simulink library "BAMLIB564xL"  (Simulink 7.3)
settings: Solver=FixedStepDiscrete  StartTime=0.0  StopTime=10.0  RelTol=1e-3
undefined symbols (not defined in the file or in its folder): CoefBuf, Kx, Ky, Order, ps32Table, s32A1, s32A2, s32ArgDcBusMsr, s32B0, s32B1, s32B2, s32C1, s32CC1, s32CC2, s32HystOff, s32HystOn, s32IntegGain, s32Kd, s32Kq, s32Lim, s32LowerLim, s32LowerLimit, s32MidId, s32MidIdx, s32ModIndex, s32OutValOff, s32OutValOn, s32PropGain, s32RampDown, s32RampUp, s32ShamOffset, s32ShamOffset1, s32ShamOffset2, s32UpperLim, s32UpperLimit, ThetaAdj, u16NSamples
(part 2 of 2)

== system BAMLIB564xL/General Functions/GFLIB_Sin ==
  note: ---------------------------------------------------------------------------------------------------------------------------------------------------------------------------------------------------
  s32In : Inport  OutDataType=fixdt(1, 16)  OutScaling=2^0
  GFLIB_Sin_SF_FLT : S-Function  FunctionName=GFLIB_Sin_SF_FLT  EnableBusSupport=off
  copyright : Subsystem
      mask Display: text(10,90,'FILE:');text(10,75,'DESRIPTION:')text(10,60,'COPYRIGHT:')text(10,45,'VERSION:')text(10,30,'DATE:')text(10,15,'AUTHOR:')
  copyright2 : Subsystem
      mask Display: text(10,90,'GFLIB_Sin_BAM_FLT.mdl');text(10,75,'sin');text(10,60,'Freescale')text(10,45,'0.1');text(10,30,'29-Sep-2010');text(10,15,'');
  logo : Subsystem
      mask Display: image(imread('logo.jpg'))
  s32Out : Outport  OutDataType=fixdt(1, 16)  OutScaling=2^0
  wires:
  GFLIB_Sin_SF_FLT/1 -> s32Out/1
  s32In/1 -> GFLIB_Sin_SF_FLT/1

== system BAMLIB564xL/General Functions/GFLIB_Sqrt ==
  note: ---------------------------------------------------------------------------------------------------------------------------------------------------------------------------------------------------
  s32In : Inport  OutDataType=fixdt(1, 16)  OutScaling=2^0
  GFLIB_Sqrt_SF_FLT : S-Function  FunctionName=GFLIB_Sqrt_SF_FLT  EnableBusSupport=off
  copyright : Subsystem
      mask Display: text(10,90,'FILE:');text(10,75,'DESRIPTION:')text(10,60,'COPYRIGHT:')text(10,45,'VERSION:')text(10,30,'DATE:')text(10,15,'AUTHOR:')
  copyright2 : Subsystem
      mask Display: text(10,90,'GFLIB_Sqrt_BAM_FLT.mdl');text(10,75,'Sqrt');text(10,60,'Freescale')text(10,45,'0.1');text(10,30,'29-Sep-2010');text(10,15,'');
  logo : Subsystem
      mask Display: image(imread('logo.jpg'))
  s32Out : Outport  OutDataType=fixdt(1, 16)  OutScaling=2^0
  wires:
  GFLIB_Sqrt_SF_FLT/1 -> s32Out/1
  s32In/1 -> GFLIB_Sqrt_SF_FLT/1

== system BAMLIB564xL/General Functions/GFLIB_Tan ==
  note: ---------------------------------------------------------------------------------------------------------------------------------------------------------------------------------------------------
  s32In : Inport  OutDataType=fixdt(1, 16)  OutScaling=2^0
  GFLIB_Tan_SF_FLT : S-Function  FunctionName=GFLIB_Tan_SF_FLT  EnableBusSupport=off
  copyright : Subsystem
      mask Display: text(10,90,'FILE:');text(10,75,'DESRIPTION:')text(10,60,'COPYRIGHT:')text(10,45,'VERSION:')text(10,30,'DATE:')text(10,15,'AUTHOR:')
  copyright2 : Subsystem
      mask Display: text(10,90,'GFLIB_Tan_BAM_FLT.mdl');text(10,75,'Tangens of argument.');text(10,60,'Freescale')text(10,45,'0.1');text(10,30,'29-Sep-2010');text(10,15,'');
  logo : Subsystem
      mask Display: image(imread('logo.jpg'))
  s32Out : Outport  OutDataType=fixdt(1, 16)  OutScaling=2^0
  wires:
  GFLIB_Tan_SF_FLT/1 -> s32Out/1
  s32In/1 -> GFLIB_Tan_SF_FLT/1

== system BAMLIB564xL/General Functions/GFLIB_UpperLimit ==
  note: ---------------------------------------------------------------------------------------------------------------------------------------------------------------------------------------------------
  s32In : Inport  OutDataType=fixdt(1, 16)  OutScaling=2^0
  GFLIB_UpperLimit_SF_FLT : S-Function  FunctionName=GFLIB_UpperLimit_SF_FLT  Parameters=s32UpperLim  EnableBusSupport=off
  copyright : Subsystem
      mask Display: text(10,90,'FILE:');text(10,75,'DESRIPTION:')text(10,60,'COPYRIGHT:')text(10,45,'VERSION:')text(10,30,'DATE:')text(10,15,'AUTHOR:')
  copyright2 : Subsystem
      mask Display: text(10,90,'GFLIB_UpperLimit_BAM_FLT.mdl');text(10,75,'Upper limit function');text(10,60,'Freescale')text(10,45,'0.1');text(10,30,'29-Sep-2010');text(10,15,'');
  logo : Subsystem
      mask Display: image(imread('logo.jpg'))
  s32Out : Outport  OutDataType=fixdt(1, 16)  OutScaling=2^0
  wires:
  GFLIB_UpperLimit_SF_FLT/1 -> s32Out/1
  s32In/1 -> GFLIB_UpperLimit_SF_FLT/1

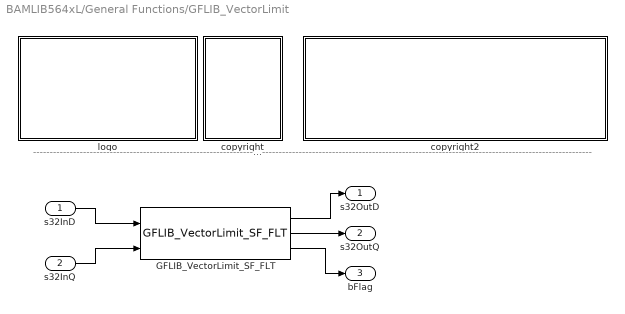
== system BAMLIB564xL/General Functions/GFLIB_VectorLimit ==
  note: ---------------------------------------------------------------------------------------------------------------------------------------------------------------------------------------------------
  s32InD : Inport  OutDataType=fixdt(1, 16)  OutScaling=2^0
  s32InQ : Inport  Port=2  OutDataType=fixdt(1, 16)  OutScaling=2^0
  GFLIB_VectorLimit_SF_FLT : S-Function  FunctionName=GFLIB_VectorLimit_SF_FLT  Parameters=s32Lim  EnableBusSupport=off
  copyright : Subsystem
      mask Display: text(10,90,'FILE:');text(10,75,'DESRIPTION:')text(10,60,'COPYRIGHT:')text(10,45,'VERSION:')text(10,30,'DATE:')text(10,15,'AUTHOR:')
  copyright2 : Subsystem
      mask Display: text(10,90,'GFLIB_VectorLimit_BAM_FLT.mdl');text(10,75,'Vector limit function');text(10,60,'Freescale')text(10,45,'0.1');text(10,30,'29-Sep-2010');text(10,15,'');
  logo : Subsystem
      mask Display: image(imread('logo.jpg'))
  s32OutD : Outport  OutDataType=fixdt(1, 16)  OutScaling=2^0
  s32OutQ : Outport  Port=2  OutDataType=fixdt(1, 16)  OutScaling=2^0
  bFlag : Outport  Port=3  OutDataType=fixdt(1, 16)  OutScaling=2^0
  wires:
  GFLIB_VectorLimit_SF_FLT/3 -> bFlag/1
  GFLIB_VectorLimit_SF_FLT/2 -> s32OutQ/1
  s32InQ/1 -> GFLIB_VectorLimit_SF_FLT/2
  GFLIB_VectorLimit_SF_FLT/1 -> s32OutD/1
  s32InD/1 -> GFLIB_VectorLimit_SF_FLT/1

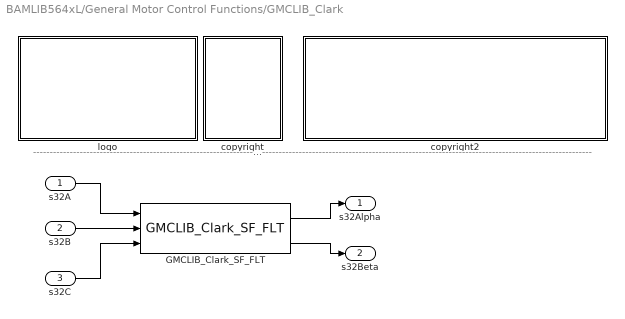
== system BAMLIB564xL/General Motor Control Functions/GMCLIB_Clark ==
  note: ---------------------------------------------------------------------------------------------------------------------------------------------------------------------------------------------------
  s32A : Inport  OutDataType=fixdt(1, 16)  OutScaling=2^0
  s32B : Inport  Port=2  OutDataType=fixdt(1, 16)  OutScaling=2^0
  s32C : Inport  Port=3  OutDataType=fixdt(1, 16)  OutScaling=2^0
  GMCLIB_Clark_SF_FLT : S-Function  FunctionName=GMCLIB_Clark_SF_FLT  EnableBusSupport=off
  copyright : Subsystem
      mask Display: text(10,90,'FILE:');text(10,75,'DESRIPTION:')text(10,60,'COPYRIGHT:')text(10,45,'VERSION:')text(10,30,'DATE:')text(10,15,'AUTHOR:')
  copyright2 : Subsystem
      mask Display: text(10,90,'GMCLIB_Clark_BAM_FLT.mdl');text(10,75,'Clarke transformation');text(10,60,'Freescale')text(10,45,'0.1');text(10,30,'29-Sep-2010');text(10,15,'');
  logo : Subsystem
      mask Display: image(imread('logo.jpg'))
  s32Alpha : Outport  OutDataType=fixdt(1, 16)  OutScaling=2^0
  s32Beta : Outport  Port=2  OutDataType=fixdt(1, 16)  OutScaling=2^0
  wires:
  GMCLIB_Clark_SF_FLT/2 -> s32Beta/1
  GMCLIB_Clark_SF_FLT/1 -> s32Alpha/1
  s32C/1 -> GMCLIB_Clark_SF_FLT/3
  s32B/1 -> GMCLIB_Clark_SF_FLT/2
  s32A/1 -> GMCLIB_Clark_SF_FLT/1

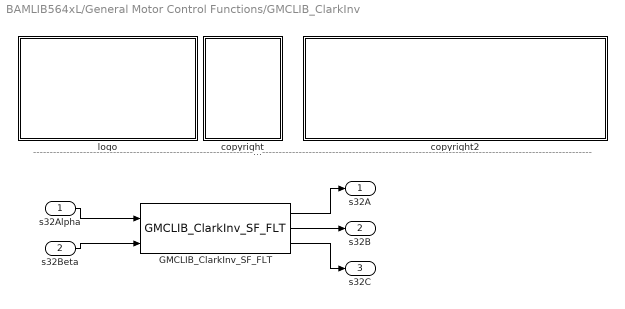
== system BAMLIB564xL/General Motor Control Functions/GMCLIB_ClarkInv ==
  note: ---------------------------------------------------------------------------------------------------------------------------------------------------------------------------------------------------
  s32Alpha : Inport  OutDataType=fixdt(1, 16)  OutScaling=2^0
  s32Beta : Inport  Port=2  OutDataType=fixdt(1, 16)  OutScaling=2^0
  GMCLIB_ClarkInv_SF_FLT : S-Function  FunctionName=GMCLIB_ClarkInv_SF_FLT  EnableBusSupport=off
  copyright : Subsystem
      mask Display: text(10,90,'FILE:');text(10,75,'DESRIPTION:')text(10,60,'COPYRIGHT:')text(10,45,'VERSION:')text(10,30,'DATE:')text(10,15,'AUTHOR:')
  copyright2 : Subsystem
      mask Display: text(10,90,'GMCLIB_ClarkInv_BAM_FLT.mdl');text(10,75,'Inverse Clarke transformation');text(10,60,'Freescale')text(10,45,'0.1');text(10,30,'29-Sep-2010');text(10,15,'');
  logo : Subsystem
      mask Display: image(imread('logo.jpg'))
  s32A : Outport  OutDataType=fixdt(1, 16)  OutScaling=2^0
  s32B : Outport  Port=2  OutDataType=fixdt(1, 16)  OutScaling=2^0
  s32C : Outport  Port=3  OutDataType=fixdt(1, 16)  OutScaling=2^0
  wires:
  GMCLIB_ClarkInv_SF_FLT/3 -> s32C/1
  GMCLIB_ClarkInv_SF_FLT/2 -> s32B/1
  GMCLIB_ClarkInv_SF_FLT/1 -> s32A/1
  s32Beta/1 -> GMCLIB_ClarkInv_SF_FLT/2
  s32Alpha/1 -> GMCLIB_ClarkInv_SF_FLT/1

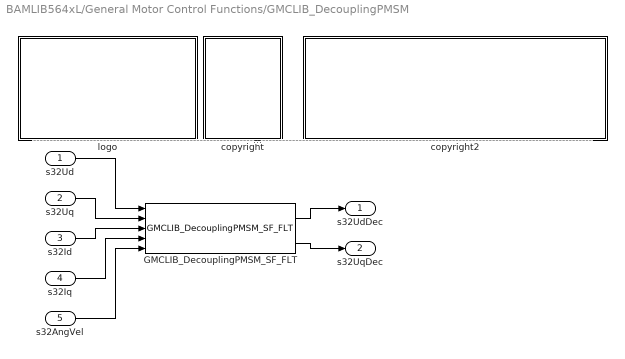
== system BAMLIB564xL/General Motor Control Functions/GMCLIB_DecouplingPMSM ==
  note: ---------------------------------------------------------------------------------------------------------------------------------------------------------------------------------------------------
  s32Ud : Inport  OutDataType=fixdt(1, 16)  OutScaling=2^0
  s32Uq : Inport  Port=2  OutDataType=fixdt(1, 16)  OutScaling=2^0
  s32Id : Inport  Port=3  OutDataType=fixdt(1, 16)  OutScaling=2^0
  s32Iq : Inport  Port=4  OutDataType=fixdt(1, 16)  OutScaling=2^0
  s32AngVel : Inport  Port=5  OutDataType=fixdt(1, 16)  OutScaling=2^0
  GMCLIB_DecouplingPMSM_SF_FLT : S-Function  FunctionName=GMCLIB_DecouplingPMSM_SF_FLT  Parameters=s32Ld,s32Lq  EnableBusSupport=off
  copyright : Subsystem
      mask Display: text(10,90,'FILE:');text(10,75,'DESRIPTION:')text(10,60,'COPYRIGHT:')text(10,45,'VERSION:')text(10,30,'DATE:')text(10,15,'AUTHOR:')
  copyright2 : Subsystem
      mask Display: text(10,90,'GMCLIB_DecouplingPMSM_BAM_FLT.mdl');text(10,75,'Decoupling of d and q axis of PMSM model.');text(10,60,'Freescale')text(10,45,'0.1');text(10,30,'29-Sep-2010');text(10,15,'');
  logo : Subsystem
      mask Display: image(imread('logo.jpg'))
  s32UdDec : Outport  OutDataType=fixdt(1, 16)  OutScaling=2^0
  s32UqDec : Outport  Port=2  OutDataType=fixdt(1, 16)  OutScaling=2^0
  wires:
  GMCLIB_DecouplingPMSM_SF_FLT/2 -> s32UqDec/1
  GMCLIB_DecouplingPMSM_SF_FLT/1 -> s32UdDec/1
  s32AngVel/1 -> GMCLIB_DecouplingPMSM_SF_FLT/5
  s32Iq/1 -> GMCLIB_DecouplingPMSM_SF_FLT/4
  s32Id/1 -> GMCLIB_DecouplingPMSM_SF_FLT/3
  s32Uq/1 -> GMCLIB_DecouplingPMSM_SF_FLT/2
  s32Ud/1 -> GMCLIB_DecouplingPMSM_SF_FLT/1

== system BAMLIB564xL/General Motor Control Functions/GMCLIB_ElimDcBusRip ==
  note: ---------------------------------------------------------------------------------------------------------------------------------------------------------------------------------------------------
  s32Alpha : Inport  OutDataType=fixdt(1, 16)  OutScaling=2^0
  s32Beta : Inport  Port=2  OutDataType=fixdt(1, 16)  OutScaling=2^0
  GMCLIB_ElimDcBusRip_SF_FLT : S-Function  FunctionName=GMCLIB_ElimDcBusRip_SF_FLT  Parameters=s32ModIndex,s32ArgDcBusMsr  EnableBusSupport=off
  copyright : Subsystem
      mask Display: text(10,90,'FILE:');text(10,75,'DESRIPTION:')text(10,60,'COPYRIGHT:')text(10,45,'VERSION:')text(10,30,'DATE:')text(10,15,'AUTHOR:')
  copyright2 : Subsystem
      mask Display: text(10,90,'GMCLIB_ElimDcBusRip_BAM_FLT.mdl');text(10,75,'DC Bus voltage ripple elimination function');text(10,60,'Freescale')text(10,45,'0.1');text(10,30,'29-Sep-2010');text(10,15,'');
  logo : Subsystem
      mask Display: image(imread('logo.jpg'))
  s32AlphaOut : Outport  OutDataType=fixdt(1, 16)  OutScaling=2^0
  s32BetaOut : Outport  Port=2  OutDataType=fixdt(1, 16)  OutScaling=2^0
  wires:
  GMCLIB_ElimDcBusRip_SF_FLT/2 -> s32BetaOut/1
  GMCLIB_ElimDcBusRip_SF_FLT/1 -> s32AlphaOut/1
  s32Beta/1 -> GMCLIB_ElimDcBusRip_SF_FLT/2
  s32Alpha/1 -> GMCLIB_ElimDcBusRip_SF_FLT/1

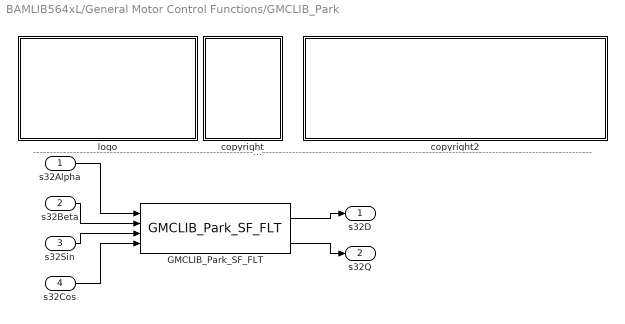
== system BAMLIB564xL/General Motor Control Functions/GMCLIB_Park ==
  note: ---------------------------------------------------------------------------------------------------------------------------------------------------------------------------------------------------
  s32Alpha : Inport  OutDataType=fixdt(1, 16)  OutScaling=2^0
  s32Beta : Inport  Port=2  OutDataType=fixdt(1, 16)  OutScaling=2^0
  s32Sin : Inport  Port=3  OutDataType=fixdt(1, 16)  OutScaling=2^0
  s32Cos : Inport  Port=4  OutDataType=fixdt(1, 16)  OutScaling=2^0
  GMCLIB_Park_SF_FLT : S-Function  FunctionName=GMCLIB_Park_SF_FLT  EnableBusSupport=off
  copyright : Subsystem
      mask Display: text(10,90,'FILE:');text(10,75,'DESRIPTION:')text(10,60,'COPYRIGHT:')text(10,45,'VERSION:')text(10,30,'DATE:')text(10,15,'AUTHOR:')
  copyright2 : Subsystem
      mask Display: text(10,90,'GMCLIB_Park_BAM_FLT.mdl');text(10,75,'Park transformation');text(10,60,'Freescale')text(10,45,'0.1');text(10,30,'29-Sep-2010');text(10,15,'');
  logo : Subsystem
      mask Display: image(imread('logo.jpg'))
  s32D : Outport  OutDataType=fixdt(1, 16)  OutScaling=2^0
  s32Q : Outport  Port=2  OutDataType=fixdt(1, 16)  OutScaling=2^0
  wires:
  GMCLIB_Park_SF_FLT/2 -> s32Q/1
  GMCLIB_Park_SF_FLT/1 -> s32D/1
  s32Cos/1 -> GMCLIB_Park_SF_FLT/4
  s32Sin/1 -> GMCLIB_Park_SF_FLT/3
  s32Beta/1 -> GMCLIB_Park_SF_FLT/2
  s32Alpha/1 -> GMCLIB_Park_SF_FLT/1

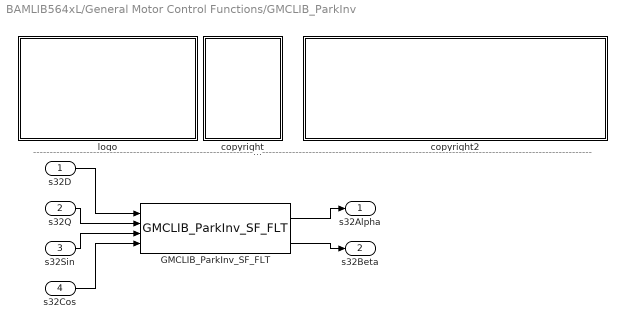
== system BAMLIB564xL/General Motor Control Functions/GMCLIB_ParkInv ==
  note: ---------------------------------------------------------------------------------------------------------------------------------------------------------------------------------------------------
  s32D : Inport  OutDataType=fixdt(1, 16)  OutScaling=2^0
  s32Q : Inport  Port=2  OutDataType=fixdt(1, 16)  OutScaling=2^0
  s32Sin : Inport  Port=3  OutDataType=fixdt(1, 16)  OutScaling=2^0
  s32Cos : Inport  Port=4  OutDataType=fixdt(1, 16)  OutScaling=2^0
  GMCLIB_ParkInv_SF_FLT : S-Function  FunctionName=GMCLIB_ParkInv_SF_FLT  EnableBusSupport=off
  copyright : Subsystem
      mask Display: text(10,90,'FILE:');text(10,75,'DESRIPTION:')text(10,60,'COPYRIGHT:')text(10,45,'VERSION:')text(10,30,'DATE:')text(10,15,'AUTHOR:')
  copyright2 : Subsystem
      mask Display: text(10,90,'GMCLIB_ParkInv_BAM_FLT.mdl');text(10,75,'Inverse Park transformation');text(10,60,'Freescale')text(10,45,'0.1');text(10,30,'29-Sep-2010');text(10,15,'');
  logo : Subsystem
      mask Display: image(imread('logo.jpg'))
  s32Alpha : Outport  OutDataType=fixdt(1, 16)  OutScaling=2^0
  s32Beta : Outport  Port=2  OutDataType=fixdt(1, 16)  OutScaling=2^0
  wires:
  GMCLIB_ParkInv_SF_FLT/2 -> s32Beta/1
  GMCLIB_ParkInv_SF_FLT/1 -> s32Alpha/1
  s32Cos/1 -> GMCLIB_ParkInv_SF_FLT/4
  s32Sin/1 -> GMCLIB_ParkInv_SF_FLT/3
  s32Q/1 -> GMCLIB_ParkInv_SF_FLT/2
  s32D/1 -> GMCLIB_ParkInv_SF_FLT/1

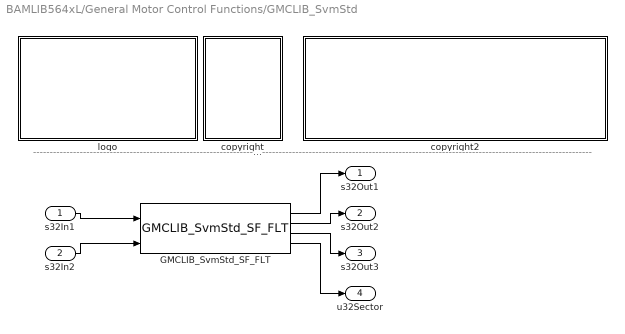
== system BAMLIB564xL/General Motor Control Functions/GMCLIB_SvmStd ==
  note: ---------------------------------------------------------------------------------------------------------------------------------------------------------------------------------------------------
  s32In1 : Inport  OutDataType=fixdt(1, 16)  OutScaling=2^0
  s32In2 : Inport  Port=2  OutDataType=fixdt(1, 16)  OutScaling=2^0
  GMCLIB_SvmStd_SF_FLT : S-Function  FunctionName=GMCLIB_SvmStd_SF_FLT  EnableBusSupport=off
  copyright : Subsystem
      mask Display: text(10,90,'FILE:');text(10,75,'DESRIPTION:')text(10,60,'COPYRIGHT:')text(10,45,'VERSION:')text(10,30,'DATE:')text(10,15,'AUTHOR:')
  copyright2 : Subsystem
      mask Display: text(10,90,'GMCLIB_SvmStd_BAM_FLT.mdl');text(10,75,'Standard Space Vector Modulation');text(10,60,'Freescale')text(10,45,'0.1');text(10,30,'29-Sep-2010');text(10,15,'');
  logo : Subsystem
      mask Display: image(imread('logo.jpg'))
  s32Out1 : Outport  OutDataType=fixdt(1, 16)  OutScaling=2^0
  s32Out2 : Outport  Port=2  OutDataType=fixdt(1, 16)  OutScaling=2^0
  s32Out3 : Outport  Port=3  OutDataType=fixdt(1, 16)  OutScaling=2^0
  u32Sector : Outport  Port=4  OutDataType=fixdt(1, 16)  OutScaling=2^0
  wires:
  GMCLIB_SvmStd_SF_FLT/4 -> u32Sector/1
  GMCLIB_SvmStd_SF_FLT/3 -> s32Out3/1
  GMCLIB_SvmStd_SF_FLT/2 -> s32Out2/1
  GMCLIB_SvmStd_SF_FLT/1 -> s32Out1/1
  s32In2/1 -> GMCLIB_SvmStd_SF_FLT/2
  s32In1/1 -> GMCLIB_SvmStd_SF_FLT/1

== system BAMLIB564xL/General Digital Filters/GDFLIB_FilterFIR/copyright ==

== system BAMLIB564xL/General Digital Filters/GDFLIB_FilterFIR/copyright2 ==

== system BAMLIB564xL/General Digital Filters/GDFLIB_FilterFIR/logo ==

== system BAMLIB564xL/General Digital Filters/GDFLIB_FilterIIR1/copyright ==

== system BAMLIB564xL/General Digital Filters/GDFLIB_FilterIIR1/copyright2 ==

== system BAMLIB564xL/General Digital Filters/GDFLIB_FilterIIR1/logo ==

== system BAMLIB564xL/General Digital Filters/GDFLIB_FilterIIR2/copyright ==

== system BAMLIB564xL/General Digital Filters/GDFLIB_FilterIIR2/copyright2 ==

== system BAMLIB564xL/General Digital Filters/GDFLIB_FilterIIR2/logo ==

== system BAMLIB564xL/General Digital Filters/GDFLIB_FilterMA/copyright ==

== system BAMLIB564xL/General Digital Filters/GDFLIB_FilterMA/copyright2 ==

== system BAMLIB564xL/General Digital Filters/GDFLIB_FilterMA/logo ==

== system BAMLIB564xL/General Functions/GFLIB_Acos/copyright ==

== system BAMLIB564xL/General Functions/GFLIB_Acos/copyright2 ==

== system BAMLIB564xL/General Functions/GFLIB_Acos/logo ==

== system BAMLIB564xL/General Functions/GFLIB_Asin/copyright ==

== system BAMLIB564xL/General Functions/GFLIB_Asin/copyright2 ==

== system BAMLIB564xL/General Functions/GFLIB_Asin/logo ==

== system BAMLIB564xL/General Functions/GFLIB_Atan/copyright ==

== system BAMLIB564xL/General Functions/GFLIB_Atan/copyright2 ==

== system BAMLIB564xL/General Functions/GFLIB_Atan/logo ==

== system BAMLIB564xL/General Functions/GFLIB_AtanYX/copyright ==

== system BAMLIB564xL/General Functions/GFLIB_AtanYX/copyright2 ==

== system BAMLIB564xL/General Functions/GFLIB_AtanYX/logo ==

== system BAMLIB564xL/General Functions/GFLIB_AtanYXShifted/copyright ==

== system BAMLIB564xL/General Functions/GFLIB_AtanYXShifted/copyright2 ==

== system BAMLIB564xL/General Functions/GFLIB_AtanYXShifted/logo ==

== system BAMLIB564xL/General Functions/GFLIB_ControllerPIp/copyright ==

== system BAMLIB564xL/General Functions/GFLIB_ControllerPIp/copyright2 ==

== system BAMLIB564xL/General Functions/GFLIB_ControllerPIp/logo ==

== system BAMLIB564xL/General Functions/GFLIB_ControllerPIpAW/copyright ==

== system BAMLIB564xL/General Functions/GFLIB_ControllerPIpAW/copyright2 ==

== system BAMLIB564xL/General Functions/GFLIB_ControllerPIpAW/logo ==

== system BAMLIB564xL/General Functions/GFLIB_ControllerPIr/copyright ==

== system BAMLIB564xL/General Functions/GFLIB_ControllerPIr/copyright2 ==

== system BAMLIB564xL/General Functions/GFLIB_ControllerPIr/logo ==

== system BAMLIB564xL/General Functions/GFLIB_ControllerPIrAW/copyright ==

== system BAMLIB564xL/General Functions/GFLIB_ControllerPIrAW/copyright2 ==

== system BAMLIB564xL/General Functions/GFLIB_ControllerPIrAW/logo ==

== system BAMLIB564xL/General Functions/GFLIB_Cos/copyright ==

== system BAMLIB564xL/General Functions/GFLIB_Cos/copyright2 ==

== system BAMLIB564xL/General Functions/GFLIB_Cos/logo ==

== system BAMLIB564xL/General Functions/GFLIB_Hyst/copyright ==

== system BAMLIB564xL/General Functions/GFLIB_Hyst/copyright2 ==

== system BAMLIB564xL/General Functions/GFLIB_Hyst/logo ==

== system BAMLIB564xL/General Functions/GFLIB_IntegratorTR/copyright ==

== system BAMLIB564xL/General Functions/GFLIB_IntegratorTR/copyright2 ==

== system BAMLIB564xL/General Functions/GFLIB_IntegratorTR/logo ==

== system BAMLIB564xL/General Functions/GFLIB_Limit/copyright ==

== system BAMLIB564xL/General Functions/GFLIB_Limit/copyright2 ==

== system BAMLIB564xL/General Functions/GFLIB_Limit/logo ==

== system BAMLIB564xL/General Functions/GFLIB_LowerLimit/copyright ==

== system BAMLIB564xL/General Functions/GFLIB_LowerLimit/copyright2 ==

== system BAMLIB564xL/General Functions/GFLIB_LowerLimit/logo ==

== system BAMLIB564xL/General Functions/GFLIB_Lut1D/copyright ==

== system BAMLIB564xL/General Functions/GFLIB_Lut1D/copyright2 ==

== system BAMLIB564xL/General Functions/GFLIB_Lut1D/logo ==

== system BAMLIB564xL/General Functions/GFLIB_Lut2D/copyright ==

== system BAMLIB564xL/General Functions/GFLIB_Lut2D/copyright2 ==

== system BAMLIB564xL/General Functions/GFLIB_Lut2D/logo ==

== system BAMLIB564xL/General Functions/GFLIB_Ramp/copyright ==

== system BAMLIB564xL/General Functions/GFLIB_Ramp/copyright2 ==

== system BAMLIB564xL/General Functions/GFLIB_Ramp/logo ==

== system BAMLIB564xL/General Functions/GFLIB_Sign/copyright ==

== system BAMLIB564xL/General Functions/GFLIB_Sign/copyright2 ==

== system BAMLIB564xL/General Functions/GFLIB_Sign/logo ==

== system BAMLIB564xL/General Functions/GFLIB_Sin/copyright ==

== system BAMLIB564xL/General Functions/GFLIB_Sin/copyright2 ==

== system BAMLIB564xL/General Functions/GFLIB_Sin/logo ==

== system BAMLIB564xL/General Functions/GFLIB_Sqrt/copyright ==

== system BAMLIB564xL/General Functions/GFLIB_Sqrt/copyright2 ==

== system BAMLIB564xL/General Functions/GFLIB_Sqrt/logo ==

== system BAMLIB564xL/General Functions/GFLIB_Tan/copyright ==

== system BAMLIB564xL/General Functions/GFLIB_Tan/copyright2 ==

== system BAMLIB564xL/General Functions/GFLIB_Tan/logo ==

== system BAMLIB564xL/General Functions/GFLIB_UpperLimit/copyright ==

== system BAMLIB564xL/General Functions/GFLIB_UpperLimit/copyright2 ==

== system BAMLIB564xL/General Functions/GFLIB_UpperLimit/logo ==

== system BAMLIB564xL/General Functions/GFLIB_VectorLimit/copyright ==

== system BAMLIB564xL/General Functions/GFLIB_VectorLimit/copyright2 ==

== system BAMLIB564xL/General Functions/GFLIB_VectorLimit/logo ==

== system BAMLIB564xL/General Motor Control Functions/GMCLIB_Clark/copyright ==

== system BAMLIB564xL/General Motor Control Functions/GMCLIB_Clark/copyright2 ==

== system BAMLIB564xL/General Motor Control Functions/GMCLIB_Clark/logo ==

== system BAMLIB564xL/General Motor Control Functions/GMCLIB_ClarkInv/copyright ==

== system BAMLIB564xL/General Motor Control Functions/GMCLIB_ClarkInv/copyright2 ==

== system BAMLIB564xL/General Motor Control Functions/GMCLIB_ClarkInv/logo ==

== system BAMLIB564xL/General Motor Control Functions/GMCLIB_DecouplingPMSM/copyright ==

== system BAMLIB564xL/General Motor Control Functions/GMCLIB_DecouplingPMSM/copyright2 ==

== system BAMLIB564xL/General Motor Control Functions/GMCLIB_DecouplingPMSM/logo ==

== system BAMLIB564xL/General Motor Control Functions/GMCLIB_ElimDcBusRip/copyright ==

== system BAMLIB564xL/General Motor Control Functions/GMCLIB_ElimDcBusRip/copyright2 ==

== system BAMLIB564xL/General Motor Control Functions/GMCLIB_ElimDcBusRip/logo ==

== system BAMLIB564xL/General Motor Control Functions/GMCLIB_Park/copyright ==

== system BAMLIB564xL/General Motor Control Functions/GMCLIB_Park/copyright2 ==

== system BAMLIB564xL/General Motor Control Functions/GMCLIB_Park/logo ==

== system BAMLIB564xL/General Motor Control Functions/GMCLIB_ParkInv/copyright ==

== system BAMLIB564xL/General Motor Control Functions/GMCLIB_ParkInv/copyright2 ==

== system BAMLIB564xL/General Motor Control Functions/GMCLIB_ParkInv/logo ==

== system BAMLIB564xL/General Motor Control Functions/GMCLIB_SvmStd/copyright ==

== system BAMLIB564xL/General Motor Control Functions/GMCLIB_SvmStd/copyright2 ==

== system BAMLIB564xL/General Motor Control Functions/GMCLIB_SvmStd/logo ==
